simulink model "simulation"  (R2015a)
settings: Solver=ode45  StartTime=0.0  StopTime=simulator.duration  RelTol=1e-3
values from neighbouring files (symbols this model uses):
  model = Model()    [main.m]    (also in simulate_fittest_individual.m)
  simulator = Simulator(model)    [main.m]    (also in simulate_fittest_individual.m)
settings Model: Creator=patrickf  LastModifiedBy=patrickf

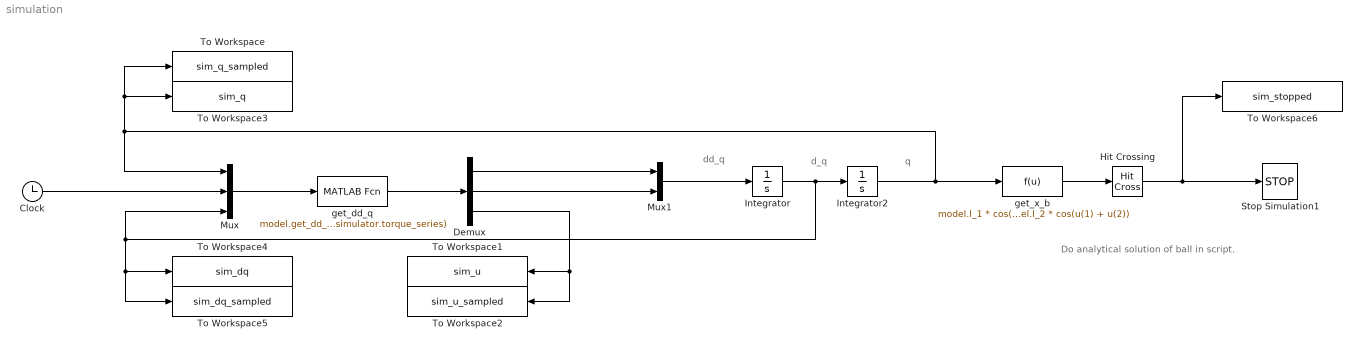
== system simulation ==
  note: Do analytical solution of ball in script.
  note: q
  note: d_q
  note: dd_q
  Clock : Clock
  Demux : Demux  Outputs=3
  Hit Crossing : HitCross
  Integrator : Integrator  InitialCondition=simulator.dq_0
  Integrator2 : Integrator  InitialCondition=simulator.q_0
  Mux : Mux  Inputs=3
  Mux1 : Mux  Inputs=2
  Stop Simulation1 : Stop
  To Workspace : ToWorkspace  VariableName=sim_q_sampled  SaveFormat=Structure With Time  SampleTime=simulator.sample_time
  To Workspace1 : ToWorkspace  VariableName=sim_u  SaveFormat=Structure With Time  SampleTime=-1
  To Workspace2 : ToWorkspace  VariableName=sim_u_sampled  SaveFormat=Structure With Time  SampleTime=simulator.sample_time
  To Workspace3 : ToWorkspace  VariableName=sim_q  SaveFormat=Structure With Time  SampleTime=-1
  To Workspace4 : ToWorkspace  VariableName=sim_dq  SaveFormat=Structure With Time  SampleTime=-1
  To Workspace5 : ToWorkspace  VariableName=sim_dq_sampled  SaveFormat=Structure With Time  SampleTime=simulator.sample_time
  To Workspace6 : ToWorkspace  VariableName=sim_stopped  SaveFormat=Structure With Time  SampleTime=-1
  get_dd_q : MATLABFcn  MATLABFcn=model.get_dd_q(u, simulator.torque_series)  OutputDimensions=3
  get_x_b : Fcn  Expr=model.l_1 * cos(u(1)) + model.l_2 * cos(u(1) + u(2))
  wires:
  Integrator/1 -> Mux/3, To Workspace5/1, To Workspace4/1, Integrator2/1
  Integrator2/1 -> Mux/1, To Workspace3/1, To Workspace/1, get_x_b/1
  Hit Crossing/1 -> To Workspace6/1, Stop Simulation1/1
  get_x_b/1 -> Hit Crossing/1
  Clock/1 -> Mux/2
  Demux/2 -> Mux1/2
  Demux/1 -> Mux1/1
  Demux/3 -> To Workspace1/1, To Workspace2/1
  Mux/1 -> get_dd_q/1
  get_dd_q/1 -> Demux/1
  Mux1/1 -> Integrator/1
